simulink model "LateralSim"  (R2018b)
settings: Solver=ode45  StartTime=0.0  StopTime=20  RelTol=1e-3
values from neighbouring files (symbols this model uses):
  initial_theta = 0    [LateralLaneKeeping.m]
  initial_x = 0    [LateralLaneKeeping.m]
  initial_y = 0    [LateralLaneKeeping.m]
undefined symbols (not defined in the file or in its folder): Rec, SDTV
libraries: vrlib x4, visionconversions x1, simulink x1, visionsinks x1
settings Model: Creator=infinity  LastModifiedBy=trey
settings DataIOCC: SaveFormat=StructureWithTime
settings OptimizationCC: LifeSpan=inf
settings DebuggingCC: LibraryContextMissingDiagnostic=none  SFExecutionAtInitializationDiag=none
settings HardwareCC: ProdBitPerSizeT=32  ProdBitPerPtrDiffT=32  ProdWordSize=32  ProdHWDeviceType=Specified
settings SFSimCC: SimUseLocalCustomCode=off
settings RTWCC: RTWUseLocalCustomCode=off
settings CodeAppCC: StateflowObjectComments=on

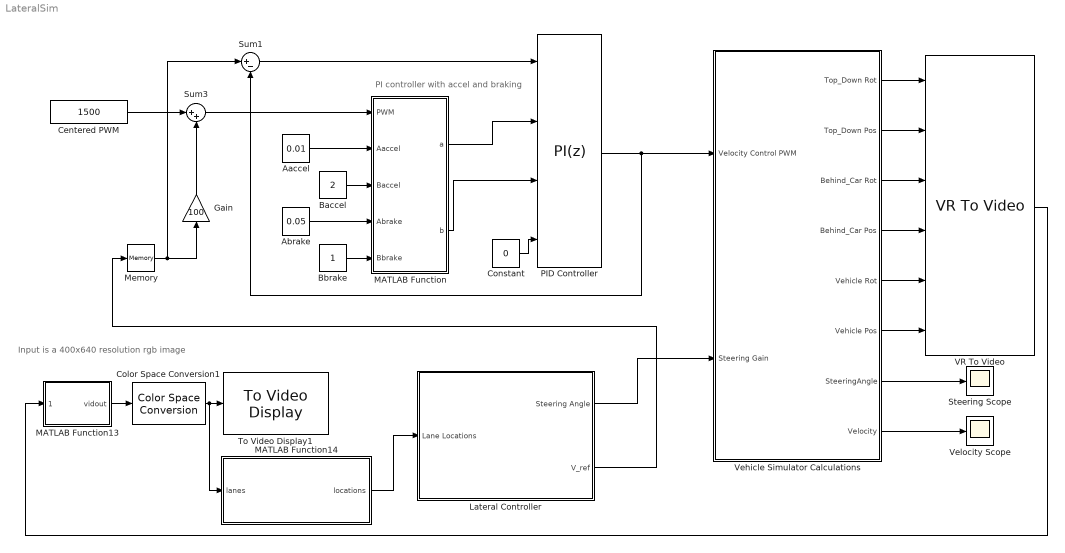
== system LateralSim ==
  note: Input is a 400x640 resolution rgb image
  note: PI controller with accel and braking
  Aaccel : Constant  Value=0.01
  Abrake : Constant  Value=0.05
  Baccel : Constant  Value=2
  Bbrake : Constant
  Centered PWM : Constant  Value=1500
  Color Space Conversion1 : visionconversions/Color Space  Conversion  conversion=Obsolete  conversionActive=R'G'B' to intensity  wp_str=D65  rec=Rec. 601 (SDTV)  sys=1125/60/2:1  imagePorts=One multidimensional signal
      settings: SourceProductName=Computer Vision System Toolbox
  Constant : Constant  Value=0
  Gain : Gain  Gain=100
  Lateral Controller : Subsystem
  MATLAB Function : MATLAB Function  TreatAsAtomicUnit=on
  MATLAB Function13 : MATLAB Function  TreatAsAtomicUnit=on
  MATLAB Function14 : MATLAB Function  TreatAsAtomicUnit=on
  Memory : Memory  InitialCondition=20
  PID Controller : simulink/Continuous/PID Controller  Controller=PI  Form=Parallel  TimeDomain=Discrete-time  SampleTime=-1  IntegratorMethod=Forward Euler  FilterMethod=Forward Euler  ControllerParametersSource=external  P=1  I=1  D=0  UseFilter=on  N=100  TunerSelectOption=Transfer Function Based (PID Tuner App)  InitialConditionSource=external  InitialConditionForIntegrator=0  InitialConditionForFilter=0  DifferentiatorICPrevScaledInput=0  ExternalReset=none  TrackingMode=off  Kt=1  LimitOutput=off  UpperSaturationLimit=inf  LowerSaturationLimit=-inf  LinearizeAsGain=on  AntiWindupMode=none  Kb=1  POutMin=[]  POutMax=[]  IOutMin=[]  IOutMax=[]  DOutMin=[]  DOutMax=[]  NOutMin=[]  NOutMax=[]  SumOutMin=[]  SumOutMax=[]  SaturationOutMin=[]  SaturationOutMax=[]  PParamMin=[]  PParamMax=[]  IParamMin=[]  IParamMax=[]  DParamMin=[]  DParamMax=[]  NParamMin=[]  NParamMax=[]  KbParamMin=[]  KbParamMax=[]  KtParamMin=[]  KtParamMax=[]  KbOutMin=[]  KbOutMax=[]  KtOutMin=[]  KtOutMax=[]  IntegratorOutMin=[]  IntegratorOutMax=[]  FilterOutMin=[]  FilterOutMax=[]  SumI1OutMin=SumI1OutMin  SumI1OutMax=SumI1OutMax  SumI2OutMin=[]  SumI2OutMax=[]  SumI3OutMin=[]  SumI3OutMax=[]  SumI4OutMin=[]  SumI4OutMax=[]  SumDOutMin=[]  SumDOutMax=[]  DifferentiatorOutMin=[]  DifferentiatorOutMax=[]  FilterDiffOutCoefMin=[]  FilterDiffOutCoefMax=[]  ReciprocalOutMin=[]  ReciprocalOutMax=[]  SumDenOutMin=[]  SumDenOutMax=[]  SumNumOutMin=[]  SumNumOutMax=[]  DivideOutMin=[]  DivideOutMax=[]  IntegratorContinuousStateAttributes=''  IntegratorStateMustResolveToSignalObject=off  IntegratorRTWStateStorageClass=Auto  FilterContinuousStateAttributes=''  FilterStateMustResolveToSignalObject=off  FilterRTWStateStorageClass=Auto  ParallelPVariant=ExternalParameters  IdealPVariant=Disabled  IVariant=ExternalParameters  DVariant=Disabled  IntegratorVariant=Discrete  SatVariant=Disabled  AWVariant=Passthrough  PCopyVariant=Disabled  TRVariant=Disabled  FdbkBlocksVariant=Forward  IdealPFdbkVariant=Disabled  SatFdbkVariant=Disabled  DerivativeFilterVariant=Disabled  NVariant=Disabled  NCopyVariant=Disabled_SignalSpec  FilterICVariant=Disabled  IntegratorICVariant=ExternalICs  ExternalResetVariant=Disabled  TRSumVariant=Passthrough  SumFdbkVariant=Disabled  SumVariant=Sum_PI
  Steering Scope : Scope
  Sum1 : Sum  Inputs=|+-
  Sum3 : Sum  Inputs=|++
  To Video Display1 : visionsinks/To Video Display  windowSizeMode=True size (1:1)  openAtMdlStart=on  fullScreen=off  videoWindowX=240  videoWindowY=191  saveWindowSize=off  videoWindowWidth=640  videoWindowHeight=400  inputColorFormat=RGB  inputType=Obsolete  imagePorts=One multidimensional signal  OutputDevice=On-screen video monitor  dataOrg=Column-major  isWindowOpen=off
      settings: SourceProductName=Computer Vision System Toolbox
  VR To Video : vrlib/VR To Video  InstantiateOnLoad=on  SampleTime=0.01  ViewEnable=on  RemoteChange=off  RemoteView=off  FieldsWritten=Top_Down.rotation.4.1.1.double#Top_Down.translation.3.1.1.double#Behind_Car.rotation.4.1.1.double#Behind_Car.translation.3.1.1.double#Vehicle.rotation.4.1.1.double#Vehicle.translation.3.1.1.double  WorldFileName=VRroadsim.wrl  WorldDescription=Lane Keeping Tester  AutoView=on  VideoDimensions=[400 640]  AllowVariableSize=off  FigureProperties="{'Position', 'Name', 'Viewpoint', 'CameraBound', 'CameraDirection', 'CameraPosition', 'CameraUpVector', 'ZoomFactor', 'Antialiasing', 'Headlight', 'Lighting', 'NavPanel', 'Sound', 'StatusBar', 'Stereo3D', 'Stereo3DCameraOffset', 'Stereo3DHIT', 'ToolBar', 'Textures', 'Transparency', 'Triad', 'Wireframe', 'NavZones', 'NavMode', 'NavSpeed', 'CaptureFileFormat', 'CaptureFileName', 'Record2DCompressMethod', 'Record2DCompressQuality', 'Record2D', 'Record2DFileName', 'Record2DFPS'; [3.0000000000000000e+01   6.0000000000000000e+01   6.4000000000000000e+02   4.0000000000000000e+02], 'Lane Keeping Tester', 'Lane Keeping Camera', 'on', [4.9979169270678331e-02   0.0000000000000000e+00  -9.9875026039496628e-01], [0.0000000000000000e+00   0.0000000000000000e+00   0.0000000000000000e+00], [0.0000000000000000e+00   1.0000000000000000e+00   0.0000000000000000e+00], [1.0000000000000000e+00], 'on', 'off', 'on', 'none', 'on', 'off', 'off', [1.0000000149011612e-01], [0.0000000000000000e+00], 'off', 'on', 'on', 'none', 'off', 'off', 'walk', 'normal', 'tif', '%f_anim_%n.tif', 'auto', [7.5000000000000000e+01], 'off', '***video***', 'auto'}"
      settings: SourceProductName=Simulink 3D Animation  SourceProductBaseCode=VR
  Vehicle Simulator Calculations : Subsystem
  Velocity Scope : Scope
  wires:
  VR To Video/1 -> MATLAB Function13/1(colordata)
  MATLAB Function13/1(vidout) -> Color Space Conversion1/1
  Color Space Conversion1/1 -> MATLAB Function14/1(lanes), To Video Display1/1
  Lateral Controller/1(Steering Angle) -> Vehicle Simulator Calculations/2(Steering Gain)
  Vehicle Simulator Calculations/1(Top_Down Rot) -> VR To Video/1
  Vehicle Simulator Calculations/2(Top_Down Pos) -> VR To Video/2
  Vehicle Simulator Calculations/3(Behind_Car Rot) -> VR To Video/3
  Vehicle Simulator Calculations/4(Behind_Car Pos) -> VR To Video/4
  Vehicle Simulator Calculations/5(Vehicle Rot) -> VR To Video/5
  Vehicle Simulator Calculations/6(Vehicle Pos) -> VR To Video/6
  Abrake/1 -> MATLAB Function/4(Abrake)
  Bbrake/1 -> MATLAB Function/5(Bbrake)
  Baccel/1 -> MATLAB Function/3(Baccel)
  Aaccel/1 -> MATLAB Function/2(Aaccel)
  MATLAB Function/1(a) -> PID Controller/2
  MATLAB Function/2(b) -> PID Controller/3
  Constant/1 -> PID Controller/4
  MATLAB Function14/1(locations) -> Lateral Controller/1(Lane Locations)
  Gain/1 -> Sum3/2
  PID Controller/1 -> Sum1/2, Vehicle Simulator Calculations/1(Velocity Control PWM)
  Sum3/1 -> MATLAB Function/1(PWM)
  Centered PWM/1 -> Sum3/1
  Memory/1 -> Gain/1, Sum1/1
  Sum1/1 -> PID Controller/1
  Lateral Controller/2(V_ref) -> Memory/1
  Vehicle Simulator Calculations/7("SteeringAngle ") -> Steering Scope/1
  Vehicle Simulator Calculations/8("Velocity ") -> Velocity Scope/1

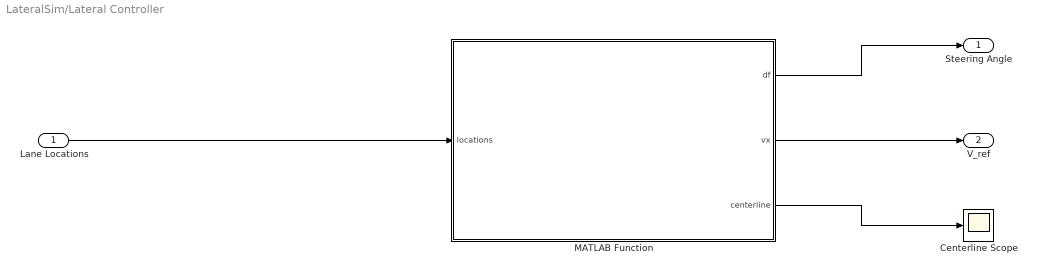
== system LateralSim/Lateral Controller ==
  Lane Locations : Inport
  Centerline Scope : Scope
  MATLAB Function : MATLAB Function  TreatAsAtomicUnit=on
  Steering Angle : Outport
  V_ref : Outport  Port=2
  wires:
  Lane Locations/1 -> MATLAB Function/1(locations)
  MATLAB Function/1(df) -> Steering Angle/1
  MATLAB Function/2(vx) -> V_ref/1
  MATLAB Function/3(centerline) -> Centerline Scope/1

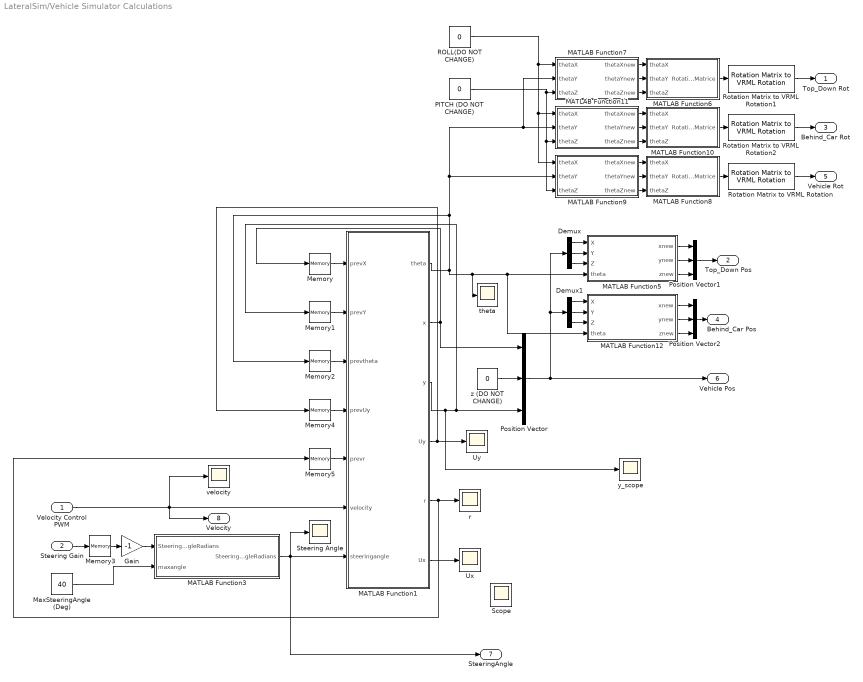
== system LateralSim/Vehicle Simulator Calculations ==
  Velocity Control PWM : Inport
  Steering Gain : Inport  Port=2
  Demux : Demux  Outputs=3
  Demux1 : Demux  Outputs=3
  Gain : Gain  Gain=-1
  MATLAB Function1 : MATLAB Function  TreatAsAtomicUnit=on
  MATLAB Function10 : MATLAB Function  TreatAsAtomicUnit=on
  MATLAB Function11 : MATLAB Function  TreatAsAtomicUnit=on
  MATLAB Function12 : MATLAB Function  TreatAsAtomicUnit=on
  MATLAB Function3 : MATLAB Function  TreatAsAtomicUnit=on
  MATLAB Function5 : MATLAB Function  TreatAsAtomicUnit=on
  MATLAB Function6 : MATLAB Function  TreatAsAtomicUnit=on
  MATLAB Function7 : MATLAB Function  TreatAsAtomicUnit=on
  MATLAB Function8 : MATLAB Function  TreatAsAtomicUnit=on
  MATLAB Function9 : MATLAB Function  TreatAsAtomicUnit=on
  MaxSteeringAngle (Deg) : Constant  Value=40
  Memory : Memory  InitialCondition=initial_x  InheritSampleTime=on
  Memory1 : Memory  InitialCondition=initial_y  InheritSampleTime=on
  Memory2 : Memory  InitialCondition=initial_theta  InheritSampleTime=on
  Memory3 : Memory  InheritSampleTime=on
  Memory4 : Memory  InheritSampleTime=on
  Memory5 : Memory  InheritSampleTime=on
  PITCH (DO NOT CHANGE) : Constant  Value=0
  Position Vector : Concatenate  NumInputs=3
  Position Vector1 : Concatenate  NumInputs=3
  Position Vector2 : Concatenate  NumInputs=3
  ROLL(DO NOT CHANGE) : Constant  Value=0
  Rotation Matrix to VRML Rotation : vrlib/Utilities/Rotation Matrix to VRML Rotation  maxzero=1e-12
      settings: SourceProductName=Simulink 3D Animation  SourceProductBaseCode=VR
  Rotation Matrix to VRML Rotation1 : vrlib/Utilities/Rotation Matrix to VRML Rotation  maxzero=1e-12
      settings: SourceProductName=Simulink 3D Animation  SourceProductBaseCode=VR
  Rotation Matrix to VRML Rotation2 : vrlib/Utilities/Rotation Matrix to VRML Rotation  maxzero=1e-12
      settings: SourceProductName=Simulink 3D Animation  SourceProductBaseCode=VR
  Scope : Scope
  Steering Angle : Scope
  Ux : Scope
  Uy : Scope
  r : Scope
  theta : Scope
  velocity : Scope
  y_scope : Scope
  z (DO NOT CHANGE) : Constant  Value=0
  Top_Down Rot : Outport
  Top_Down Pos : Outport  Port=2
  Behind_Car Rot : Outport  Port=3
  Behind_Car Pos : Outport  Port=4
  Vehicle Rot : Outport  Port=5
  Vehicle Pos : Outport  Port=6
  "SteeringAngle " : Outport  Port=7
  "Velocity " : Outport  Port=8
  wires:
  MATLAB Function9/2(thetaYnew) -> MATLAB Function8/2(thetaY)
  MATLAB Function12/2(ynew) -> Position Vector2/2
  MATLAB Function1/1(theta) -> theta/1, MATLAB Function12/4(theta), MATLAB Function5/4(theta), MATLAB Function11/2(thetaY), MATLAB Function7/2(thetaY), MATLAB Function9/2(thetaY), Memory2/1
  ROLL(DO NOT CHANGE)/1 -> MATLAB Function9/1(thetaX), MATLAB Function11/1(thetaX), MATLAB Function7/1(thetaX)
  Demux/1 -> MATLAB Function5/1(X)
  MATLAB Function10/1(RotationMatrice) -> Rotation Matrix to VRML Rotation2/1
  Demux/3 -> MATLAB Function5/3(Z)
  MATLAB Function1/2(x) -> Position Vector/1, Memory/1
  Position Vector2/1 -> Behind_Car Pos/1
  MATLAB Function5/2(ynew) -> Position Vector1/2
  MATLAB Function1/3(y) -> y_scope/1, Memory1/1, Position Vector/3
  MATLAB Function9/3(thetaZnew) -> MATLAB Function8/3(thetaZ)
  MATLAB Function7/2(thetaYnew) -> MATLAB Function6/2(thetaY)
  MATLAB Function8/1(RotationMatrice) -> Rotation Matrix to VRML Rotation/1
  MATLAB Function5/1(xnew) -> Position Vector1/1
  MATLAB Function7/1(thetaXnew) -> MATLAB Function6/1(thetaX)
  MATLAB Function9/1(thetaXnew) -> MATLAB Function8/1(thetaX)
  MATLAB Function12/1(xnew) -> Position Vector2/1
  MATLAB Function11/1(thetaXnew) -> MATLAB Function10/1(thetaX)
  MATLAB Function6/1(RotationMatrice) -> Rotation Matrix to VRML Rotation1/1
  Rotation Matrix to VRML Rotation/1 -> Vehicle Rot/1
  MATLAB Function11/3(thetaZnew) -> MATLAB Function10/3(thetaZ)
  Demux/2 -> MATLAB Function5/2(Y)
  MATLAB Function5/3(znew) -> Position Vector1/3
  MATLAB Function12/3(znew) -> Position Vector2/3
  Demux1/1 -> MATLAB Function12/1(X)
  Position Vector/1 -> Demux/1, Demux1/1, Vehicle Pos/1
  Demux1/3 -> MATLAB Function12/3(Z)
  PITCH (DO NOT CHANGE)/1 -> MATLAB Function11/3(thetaZ), MATLAB Function9/3(thetaZ), MATLAB Function7/3(thetaZ)
  MATLAB Function11/2(thetaYnew) -> MATLAB Function10/2(thetaY)
  Demux1/2 -> MATLAB Function12/2(Y)
  MATLAB Function7/3(thetaZnew) -> MATLAB Function6/3(thetaZ)
  Rotation Matrix to VRML Rotation1/1 -> Top_Down Rot/1
  z (DO NOT CHANGE)/1 -> Position Vector/2
  Rotation Matrix to VRML Rotation2/1 -> Behind_Car Rot/1
  Steering Gain/1 -> Memory3/1
  MATLAB Function3/1(SteeringAngleRadians) -> "SteeringAngle "/1, MATLAB Function1/7(steeringangle), Steering Angle/1
  Position Vector1/1 -> Top_Down Pos/1
  MATLAB Function1/4(Uy) -> Uy/1, Memory4/1
  MATLAB Function1/5(r) -> Memory5/1, r/1
  Memory4/1 -> MATLAB Function1/4(prevUy)
  Memory5/1 -> MATLAB Function1/5(prevr)
  Memory2/1 -> MATLAB Function1/3(prevtheta)
  Memory1/1 -> MATLAB Function1/2(prevY)
  Memory/1 -> MATLAB Function1/1(prevX)
  MaxSteeringAngle (Deg)/1 -> MATLAB Function3/2(maxangle)
  Memory3/1 -> Gain/1
  Gain/1 -> MATLAB Function3/1("SteeringAngleRadians ")
  Velocity Control PWM/1 -> MATLAB Function1/6(velocity), velocity/1, "Velocity "/1
  MATLAB Function1/6(Ux) -> Ux/1
  ? -> Scope/1

== matlab function LateralSim/Vehicle Simulator Calculations/MATLAB Function1 ==
  data: theta output; x output; y output; prevX input; prevY input; prevtheta input; prevUy input; prevr input; velocity input; steeringangle input; Uy output; r output; Ux output
function [theta, x, y, Uy, r, Ux] = POSupdate(prevX,prevY,prevtheta,prevUy,prevr,velocity,steeringangle)
% Vehicle Parameters
m = 1650;
Iz = 2235;
L = 2.47;
a = 0.43*L;
b = L-a;

% Define tire parameters
frontTire.Ca = 200000;
frontTire.Fz = (b/L)*m*9.8;
frontTire.muP = 1;
frontTire.muS = .8;

rearTire.Ca = 200000;
rearTire.Fz = (a/L)*m*9.8;
rearTire.muP = 1.1;
rearTire.muS = .9;

%%
% Set the time step, simulation time and number of points
tstep = 0.01;

% Ux = velocity; %forward velocity

Ux = velocity;
delta = -1*steeringangle;

% Solve for alphaf, alphar given Ux, delta, r and Uy
alphaf = (prevUy+a*prevr)/Ux - delta;
alphar = (prevUy-b*prevr)/Ux;

% Solve for Fyf and Fyr
Fyf = -frontTire.Ca*alphaf;
Fyr = -rearTire.Ca*alphar;

% Solve for derivatives drdt dUydt
drdt = (a*Fyf-b*Fyr)/Iz;
dUydt = (Fyf + Fyr)/m - prevr*Ux;

% Update time and states
Uy = prevUy + tstep*dUydt; %lateral velocity
r = prevr + tstep*drdt; % yaw rate

%% Position Calculation

theta = -1*(r*tstep)+prevtheta;
velmag = sqrt((Ux*tstep)^2+(Uy*tstep)^2);
x = prevX + velmag*cos(theta);
y = prevY + velmag*sin(theta);

if velocity < 7
    directionalmagnitude = velocity * tstep;
    theta = steeringangle/20+prevtheta;
    x = prevX + directionalmagnitude*cos(theta);
    y = prevY + directionalmagnitude*sin(theta);
end

== matlab function LateralSim/MATLAB Function ==
  data: PWM input; a output; b output; Aaccel input; Baccel input; Abrake input; Bbrake input
function [a,b] = AccelBrake(PWM,Aaccel,Baccel,Abrake,Bbrake)
if PWM > 1500
    % Acceleration values
    a = Aaccel;
    b = Baccel;
else
    % Braking values
    a = Abrake;
    b = Bbrake;
end

== matlab function LateralSim/Lateral Controller/MATLAB Function ==
  data: df output; locations input [..256000]; vx output; centerline output
function [df,vx, centerline]= fcn(locations)

vx = 20;

% The locatoins data has three vertically stacked copies of the lane
% locations because we get this data from each of the RGB channels
divthree = (length(locations)/3);
trimmed_locations = locations(1:divthree,:);
trimmed_locations_x = trimmed_locations(:, 1);
trimmed_locations_y = trimmed_locations(:, 2);

% now we get the coordinate of the left and right lane at the botom of the
% frame, the left lane is at y_max and the right lane is at y_min
% x_min = min(trimmed_locations_x);
y_min = min(trimmed_locations_y);

% x_max = max(trimmed_locations_x);
y_max = max(trimmed_locations_y);

left_lane = y_max;
right_lane = y_min;

centerline = (left_lane + right_lane)/2;

kp = 2;

% df should be an angle output in radians
df = deg2rad(kp*(centerline));

% df = deg2rad(0);

% Note
% turning right is negative radians

% Questions
% - What is this locations array, do I have access to all elements of it or
% do they arrive at each loop, how are they labeled I'm confused by the pdf
% - What setpoint am I aiming for?
% - If I set steering to 0, the road never goes away, is this just a
% perfectly straight road? Why would it be that way
% displaying locations in this function, I see that they jump around wildly
% while the video shows two stagnant lane lines, what gives...

== matlab function LateralSim/Vehicle Simulator Calculations/MATLAB Function3 ==
  data: SteeringAngleRadians input; SteeringAngleRadians output; maxangle input
function SteeringAngleRadians = steeringanglemax(SteeringAngleRadians,maxangle)

if abs(SteeringAngleRadians) >= deg2rad(maxangle)
    SteeringAngleRadians = deg2rad(maxangle);
end

== matlab function LateralSim/Vehicle Simulator Calculations/MATLAB Function5 ==
  data: xnew output; ynew output; znew output; X input; Y input; Z input; theta input
function [xnew,ynew,znew] = POSCamera(X,Y,Z,theta)

offsetxref = 15;
offsetzref = -2;

xnew = X + offsetxref*cos(theta) - offsetzref*sin(theta);
ynew = Y + 10;
znew = Z + offsetxref*sin(theta) + offsetzref*cos(theta);

== matlab function LateralSim/Vehicle Simulator Calculations/MATLAB Function6 ==
  data: thetaX input; RotationMatrice output; thetaY input; thetaZ input
function RotationMatrice = rotat3(thetaX, thetaY, thetaZ)
RotationMatrice = [cos(thetaY)*cos(thetaZ);-cos(thetaY)*sin(thetaZ);sin(thetaY);...
    cos(thetaX)*sin(thetaZ)+sin(thetaX)*sin(thetaY)*cos(thetaZ);cos(thetaX)*cos(thetaZ)-sin(thetaX)*sin(thetaY)*sin(thetaZ);-sin(thetaX)*cos(thetaY);...
    sin(thetaX)*sin(thetaZ)-cos(thetaX)*sin(thetaY)*cos(thetaZ);sin(thetaX)*cos(thetaZ)+cos(thetaX)*sin(thetaY)*sin(thetaZ);cos(thetaX)*cos(thetaY)];

== matlab function LateralSim/Vehicle Simulator Calculations/MATLAB Function7 ==
  data: thetaX input; thetaXnew output; thetaY input; thetaZ input; thetaYnew output; thetaZnew output
function [thetaXnew, thetaYnew, thetaZnew] = offset(thetaX,thetaY,thetaZ)

thetaXnew = thetaX + pi/2 - pi/8;
thetaYnew = thetaY + pi/2;
thetaZnew = thetaZ;

== matlab function LateralSim/Vehicle Simulator Calculations/MATLAB Function8 ==
  data: thetaX input; RotationMatrice output; thetaY input; thetaZ input
function RotationMatrice = rotat3(thetaX, thetaY, thetaZ)
RotationMatrice = [cos(thetaY)*cos(thetaZ);-cos(thetaY)*sin(thetaZ);sin(thetaY);...
    cos(thetaX)*sin(thetaZ)+sin(thetaX)*sin(thetaY)*cos(thetaZ);cos(thetaX)*cos(thetaZ)-sin(thetaX)*sin(thetaY)*sin(thetaZ);-sin(thetaX)*cos(thetaY);...
    sin(thetaX)*sin(thetaZ)-cos(thetaX)*sin(thetaY)*cos(thetaZ);sin(thetaX)*cos(thetaZ)+cos(thetaX)*sin(thetaY)*sin(thetaZ);cos(thetaX)*cos(thetaY)];

== matlab function LateralSim/Vehicle Simulator Calculations/MATLAB Function9 ==
  data: thetaX input; thetaXnew output; thetaY input; thetaZ input; thetaYnew output; thetaZnew output
function [thetaXnew, thetaYnew, thetaZnew] = offset(thetaX,thetaY,thetaZ)

thetaXnew = thetaX + 0;
thetaYnew = thetaY - pi/2;
thetaZnew = thetaZ + 0;

== matlab function LateralSim/Vehicle Simulator Calculations/MATLAB Function10 ==
  data: thetaX input; RotationMatrice output; thetaY input; thetaZ input
function RotationMatrice = rotat3(thetaX, thetaY, thetaZ)
RotationMatrice = [cos(thetaY)*cos(thetaZ);-cos(thetaY)*sin(thetaZ);sin(thetaY);...
    cos(thetaX)*sin(thetaZ)+sin(thetaX)*sin(thetaY)*cos(thetaZ);cos(thetaX)*cos(thetaZ)-sin(thetaX)*sin(thetaY)*sin(thetaZ);-sin(thetaX)*cos(thetaY);...
    sin(thetaX)*sin(thetaZ)-cos(thetaX)*sin(thetaY)*cos(thetaZ);sin(thetaX)*cos(thetaZ)+cos(thetaX)*sin(thetaY)*sin(thetaZ);cos(thetaX)*cos(thetaY)];

== matlab function LateralSim/Vehicle Simulator Calculations/MATLAB Function11 ==
  data: thetaX input; thetaXnew output; thetaY input; thetaZ input; thetaYnew output; thetaZnew output
function [thetaXnew, thetaYnew, thetaZnew] = offset(thetaX,thetaY,thetaZ)

thetaXnew = thetaX + pi/8;
thetaYnew = thetaY + pi/2;
thetaZnew = thetaZ;

== matlab function LateralSim/Vehicle Simulator Calculations/MATLAB Function12 ==
  data: xnew output; ynew output; znew output; X input; Y input; Z input; theta input
function [xnew,ynew,znew] = POSCamera(X,Y,Z,theta)

offsetxref = -5;
offsetzref = -2;

xnew = X + offsetxref*cos(theta) - offsetzref*sin(theta);
ynew = Y + 10;
znew = Z + offsetxref*sin(theta) + offsetzref*cos(theta);

== matlab function LateralSim/MATLAB Function13 ==
  data: colordata input; vidout output
function vidout = colorfind(colordata)

rdesired = 206;
gdesired = 206;
bdesired = 41;

for i = 1:400
    for j = 1:640
        if colordata(i,j,1) == rdesired &&...
                colordata(i,j,2) == gdesired &&...
                colordata(i,j,3) == bdesired
            colordata(i,j,1) = 255;
        else
            colordata(i,j,1) = 0;
            colordata(i,j,2) = 0;
            colordata(i,j,3) = 0;
        end
    end
end

vidout = colordata;

== matlab function LateralSim/MATLAB Function14 ==
  data: lanes input; locations output size=[256000 2] [0..256000]
function locations = LaneLocations(lanes)
width = 8;%meters
height = 5;%meters
offset = -0.3;
pixelsize = width/640; %m/pixel
locations = [0,0;0 0];
[x_pixel,y_pixel] = find(fliplr(lanes') ~= 0);
coder.varsize('locations',[256000 2]);
x_inertial = y_pixel.*pixelsize;
y_inertial = x_pixel.*pixelsize-width/2-offset;
locations = [x_inertial,y_inertial]; %m
